simulink model "tests_model"  (R2025b)
settings: Solver=FixedStepDiscrete  StartTime=0.0  StopTime=inf  FixedStep=0.01  RelTol=1e-3
libraries: dspnetwork x1
settings Model: NumberOfSteps=10  Creator=Gabriel  LastModifiedBy=henri
settings SFSimCC: SimCustomInitializer=SS_App_Init();  SimUserIncludeDirs=..\..\include
settings SFSimCC: SimCustomHeaderCode=|
  | #include "ss_app.h"
  | 
  | #include "ss_input_proc.h"
  | 
  | #include "ss_operation.h"
  | 
  | #include "ss_types.h"
  | 
  | #include "ss_calib.h"
  | 
  | #include "ss_timer.h"
  | 
  | #include "ss_inhibit_safety_conditions.h"
  | 
  | #include "co2.h"
  | 
  | #include "ss_fuel.h"
  | 
  | #include "ss_control.h"
settings SFSimCC: SimUserSources=|
  | ..\..\src\ss_operation.c
  | 
  | ..\..\src\ss_input_proc.c
  | 
  | ..\..\src\ss_app.c
  | 
  | ..\..\src\timer.c
  | 
  | ..\..\src\ss_inhibit_safety_conditions.c
  | 
  | ..\..\src\co2.c
  | 
  | ..\..\src\ss_control.c
  | 
  | ..\..\src\ss_fuel.c

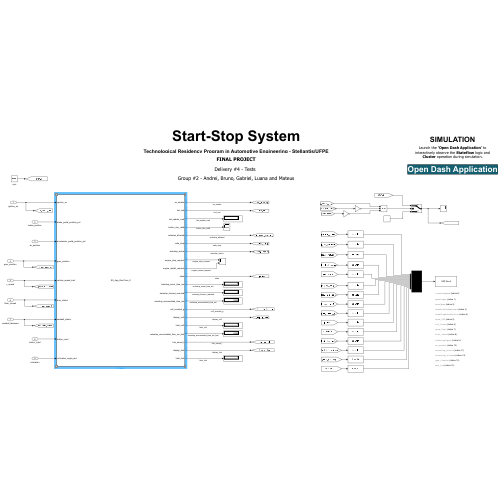
[thumbnail: Simulink's stored preview of the top-level diagram]
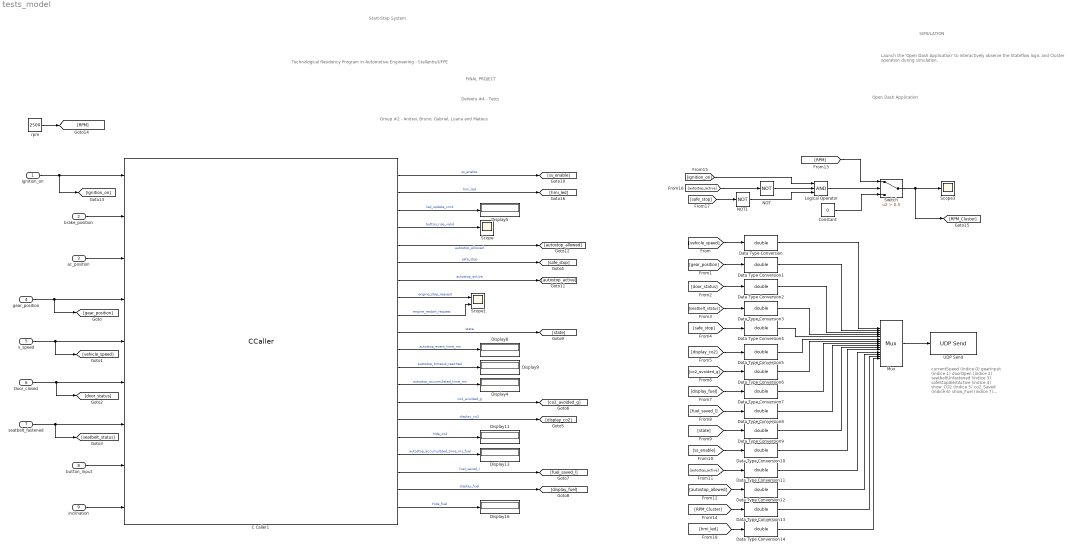
== system tests_model ==
  note: currentSpeed (índice 0)
      | gearInput (índice 1)
      | doorOpen (índice 2)
      | seatbeltUnfastened (índice 3)
      | safeStopAlertActive (índice 4)
      | show_CO2 (índice 5)
      | co2_Saved (índice 6)
      | show_Fuel (índice 7)
      | fuel_Saved (índice 8)
      | ssStatusInput (índice 9)
      | ss_enable (índice 10)
      |
      | autostop_active (índice 11)
      | autostop_allowed (índice 12)
      | rpm_cluster (índice 13)
      | hmi_led (índice 14)
  note: Open Dash Application
  note: Technological Residency Program in Automotive Engineering - Stellantis/UFPE
  note: Start-Stop System
  note: FINAL PROJECT
  note: Group #2 - Andrei, Bruno, Gabriel, Luana and Mateus
  note: Delivery #4 - Tests
  note: SIMULATION
  note: Launch the 'Open Dash Application' to interactively observe the Stateflow logic and Cluster operation during simulation.
  ignition_on : Inport
  brake_position : Inport  Port=2
  ac_position : Inport  Port=3
  gear_position : Inport  Port=4
  v_speed : Inport  Port=5
  Door_closed : Inport  Port=6
  seatbelt_fastened : Inport  Port=7
  button_input : Inport  Port=8
  inclination : Inport  Port=9
  C Caller1 : CCaller  FunctionName=SS_App_Run10ms_If  PortSpecificationStruct="%)30     .    ^#,   8    (     @         %    \"    !T    !     0         %  0 \"0    $    _    07)G3F%M90  4&]R=$YA;64 4V-O<&4     26YD97@     5'EP90      4VEZ90      27-';&]B86P   X   !     !@    @    $          4    (     0    L    !         !     +    :6=N:71I;VY?;VX       X   !     !@    @    $          4    (     0    L    !         !     +    :6=N:71I;VY?;VX       X    X    !@    @    $     ...(+17556 chars)"  SampleTime=0.01
  Constant : Constant  Value=0
  Data Type Conversion{,1..14} (15 alike) : DataTypeConversion  OutDataTypeStr=double  SaturateOnIntegerOverflow=off  RndMeth=Floor
  Display{4..5,8..9,11,13,16} (7 alike) : Display
  Logical Operator : Logic  Inputs=3  AllPortsSameDT=off  OutDataTypeStr=boolean
  Mux : Mux  Inputs=15
  NOT : Logic  Operator=NOT  IconShape=distinctive  AllPortsSameDT=off  OutDataTypeStr=boolean
  NOT1 : Logic  Operator=NOT  IconShape=distinctive  AllPortsSameDT=off  OutDataTypeStr=boolean
  Scope : Scope
      settings: ActiveDisplayYMinimum=-1.3720535825056084  ActiveDisplayYMaximum=4.2527611164993893
  Scope1 : Scope  NumInputPorts=2
      settings: ActiveDisplayYMinimum=-1.3720535825056084  ActiveDisplayYMaximum=4.2527611164993893
  Scope3 : Scope
      settings: DataLoggingVariableName=ScopeData3
  Switch : Switch  Criteria=u2 > Threshold  Threshold=0.5  SaturateOnIntegerOverflow=off  InputSameDT=off
  UDP Send : dspnetwork/UDP Send  remoteURL='127.0.0.1'  remotePort=55000  localURL='0.0.0.0'  localPortSource=Automatically determine  localPort=-1  sendBufferSize=8192  sampletime=-1  blockPlatform=[]  separateLengthPort=0
      settings: LibrarySourceBlock=dspsnks4/UDP Send
  rpm : Constant  Value=2500  OutDataTypeStr=double
  wires:
  ignition_on/1 -> C Caller1/1, [ignition_on]
  C Caller1/1 -> [ss_enable]  "ss_enable"
  C Caller1/2 -> [hmi_led]  "hmi_led"
  C Caller1/4 -> Scope/1  "button_rise_valid"
  C Caller1/6 -> [safe_stop]  "safe_stop"
  C Caller1/3 -> Display5/1  "led_update_cmd"
  C Caller1/7 -> [autostop_active]  "autostop_active"
  C Caller1/8 -> Scope1/1  "engine_stop_request"
  C Caller1/9 -> Scope1/2  "engine_restart_request"
  C Caller1/10 -> [state]  "state"
  C Caller1/11 -> Display8/1  "autostop_event_time_ms"
  C Caller1/12 -> Display9/1  "autostop_timeout_reached"
  brake_position/1 -> C Caller1/2
  ac_position/1 -> C Caller1/3
  gear_position/1 -> [gear_position], C Caller1/4
  v_speed/1 -> [vehicle_speed], C Caller1/5
  Door_closed/1 -> [door_status], C Caller1/6
  seatbelt_fastened/1 -> [seatbelt_status], C Caller1/7
  button_input/1 -> C Caller1/8
  inclination/1 -> C Caller1/9
  C Caller1/13 -> Display4/1  "autostop_accumulated_time_ms"
  C Caller1/14 -> [co2_avoided_g]  "co2_avoided_g"
  C Caller1/15 -> [display_co2]  "display_co2"
  C Caller1/16 -> Display11/1  "hide_co2"
  C Caller1/5 -> [autostop_allowed]  "autostop_allowed"
  C Caller1/17 -> Display13/1  "autostop_accumulated_time_ms_fuel"
  C Caller1/18 -> [fuel_saved_l]  "fuel_saved_l"
  C Caller1/19 -> [display_fuel]  "display_fuel"
  C Caller1/20 -> Display16/1  "hide_fuel"
  [vehicle_speed] -> Data Type Conversion/1
  [gear_position] -> Data Type Conversion1/1
  [door_status] -> Data Type Conversion2/1
  [seatbelt_status] -> Data Type Conversion3/1
  [safe_stop] -> Data Type Conversion4/1
  [display_co2] -> Data Type Conversion5/1
  [co2_avoided_g] -> Data Type Conversion6/1
  [display_fuel] -> Data Type Conversion7/1
  [fuel_saved_l] -> Data Type Conversion8/1
  [state] -> Data Type Conversion9/1
  Data Type Conversion/1 -> Mux/1
  Data Type Conversion1/1 -> Mux/2
  Data Type Conversion2/1 -> Mux/3
  Data Type Conversion3/1 -> Mux/4
  Data Type Conversion4/1 -> Mux/5
  Data Type Conversion5/1 -> Mux/6
  Data Type Conversion6/1 -> Mux/7
  Data Type Conversion7/1 -> Mux/8
  Data Type Conversion8/1 -> Mux/9
  Data Type Conversion9/1 -> Mux/10
  Mux/1 -> UDP Send/1
  Data Type Conversion10/1 -> Mux/11
  [ss_enable] -> Data Type Conversion10/1
  Data Type Conversion11/1 -> Mux/12
  [autostop_active] -> Data Type Conversion11/1
  Data Type Conversion12/1 -> Mux/13
  [autostop_allowed] -> Data Type Conversion12/1
  Switch/1 -> [RPM_Cluster], Scope3/1
  Constant/1 -> Switch/3
  [ignition_on] -> Logical Operator/1
  [autostop_active] -> NOT/1
  [safe_stop] -> NOT1/1
  NOT/1 -> Logical Operator/2
  NOT1/1 -> Logical Operator/3
  Logical Operator/1 -> Switch/2
  rpm/1 -> [RPM]
  [RPM] -> Switch/1
  Data Type Conversion13/1 -> Mux/14
  [RPM_Cluster] -> Data Type Conversion13/1
  Data Type Conversion14/1 -> Mux/15
  [hmi_led] -> Data Type Conversion14/1
